simulink model "ModeAdjust"  (R2018b)
settings: Solver=FixedStepDiscrete  StartTime=0.0  StopTime=inf  FixedStep=0.01  RelTol=1e-3
undefined symbols (not defined in the file or in its folder): IfKeSMSbSeatMovBkRclnEnable_Val, IfKeSMSbSeatMovFrwdBkwdEnable_Val, IfKeSMSbSeatMovFtrstEnable_Val, IfKeSMSbSeatMovHdrstFrwdBkwdEnable_Val, IfKeSMSbSeatMovHdUpwdDnwdEnable_Val, IfKeSMSbSeatMovLgrstEnable_Val, IfKeSMSbSeatMovLtwdRtwdEnable_Val, IfVeSMSeStNumConfig, KeSMSbArmscreenMovEnable_Val, KeSMSbSeatMovLgrstExpdEnable_Val, KeSMSuFirstRwStBackPosDelta_Val, KeSMSuFirstRwStBackPosTolr_Val, KeSMSuFirstRwStCushFrntPosDelta_Val, KeSMSuFirstRwStCushFrntPosTolr_Val, KeSMSuFirstRwStCushRePosDelta_Val, KeSMSuFirstRwStCushRePosTolr_Val, KeSMSuFirstRwStFootrestPosDelta_Val, KeSMSuFirstRwStFootrestPosTolr_Val, KeSMSuFirstRwStFwdBkwdPosDelta_Val, KeSMSuFirstRwStFwdBkwdPosTolr_Val, KeSMSuMdMotFinshdTm_Val, KeSMSuMdRetryTm1_Val, KeSMSuModeReqDurgTm_Val, KeSMSuSecRwStArmTochPosDelta_Val, KeSMSuSecRwStArmTochPosTolr_Val, KeSMSuSecRwStBackPosDelta_Val, KeSMSuSecRwStBackPosTolr_Val, KeSMSuSecRwStFtrstUpwdDnwdPosDelta_Val, KeSMSuSecRwStFtrstUpwdDnwdPosTolr_Val, KeSMSuSecRwStFwdBkwdPosDelta_Val, KeSMSuSecRwStFwdBkwdPosTolr_Val, KeSMSuSecRwStHeadrestFwdBkwdPosDelta_Val, KeSMSuSecRwStHeadrestFwdBkwdPosTolr_Val, KeSMSuSecRwStHeadrestUpwdDwnwdPosDelta_Val, KeSMSuSecRwStHeadrestUpwdDwnwdPosTolr_Val, KeSMSuSecRwStLegrestInOutPosDelta_Val, KeSMSuSecRwStLegrestInOutPosTolr_Val, KeSMSuSecRwStLegrestUpwdDwnwdPosDelta_Val, KeSMSuSecRwStLegrestUpwdDwnwdPosTolr_Val, KeSMSuSecRwStLwdRwdPosDelta_Val, KeSMSuSecRwStLwdRwdPosTolr_Val, KeSMSuSecRwStVIPFtrstRefAngle_Val, KeSMSuThirdRwStFwdBkwdPosDelta_Val, KeSMSuThirdRwStFwdBkwdPosTolr_Val, KeSMSuThrdRwCushFoldPosDelta_Val, KeSMSuThrdRwCushFoldPosTolr_Val, KeSMSuThrdRwStBackPosDelta_Val, KeSMSuThrdRwStBackPosTolr_Val, KeSMSw4SLegrstCloseMdSecRwLtStFtrstUpwdDnwdPos_Val, KeSMSw4SLegrstCloseMdSecRwLtStFtrstUpwdDnwdPosMax_Val, KeSMSw4SLegrstCloseMdSecRwLtStFtrstUpwdDnwdPosMin_Val, KeSMSw4SLegrstCloseMdSecRwLtStLgrstOtwdInwdPos_Val, KeSMSw4SLegrstCloseMdSecRwLtStLgrstOtwdInwdPosMax_Val, KeSMSw4SLegrstCloseMdSecRwLtStLgrstOtwdInwdPosMin_Val, KeSMSw4SLegrstCloseMdSecRwLtStLgrstUpwdDnwdPos_Val, KeSMSw4SLegrstCloseMdSecRwLtStLgrstUpwdDnwdPosMax_Val, KeSMSw4SLegrstCloseMdSecRwLtStLgrstUpwdDnwdPosMin_Val, KeSMSw4SLegrstCloseMdSecRwRtStFtrstUpwdDnwdPos_Val, KeSMSw4SLegrstCloseMdSecRwRtStFtrstUpwdDnwdPosMax_Val, KeSMSw4SLegrstCloseMdSecRwRtStFtrstUpwdDnwdPosMin_Val ... (+1138)
libraries: Lib x401
(part 29 of 35)

== system ModeAdjust/ModeAdjustRunnable_sys/ModeAdjust/ArrivedAtTargetPosChk/Ly/R2Rt ==
  SecRwLtStsPoss : Inport
  ModeStCalib_2L : Inport  Port=2
  StConfig : Inport  Port=3
  SecRwLtStsPoss4s : Inport  Port=4
  StConfig4s : Inport  Port=5
  SecRwRtStPossV : Inport  Port=6
  PosV4s : Inport  Port=7
  Rt4sHightIndex : Inport  Port=8
  PosDeltaCalib : Inport  Port=9
  Bus Creator{,1..6} (7 alike) : BusCreator  Inputs=9
  Bus Selector : BusSelector  OutputSignals=IfVeSMSuSecRwRtStBkReclnUpwdDnwdPos_Val_read,IfVeSMSuSecRwRtStFrwdBkwdPos_Val_read,IfVeSMSuSecRwRtStHPassStUpwdDnwdPos_Val_read,IfVeSMSuSecRwRtStLgrstUpwdDnwdPos_Val_read,IfVeSMSuSecRwRtStLtwdRtwdPos_Val_read,SecRwRtStArmScrnPos_Val_read
  Bus Selector1 : BusSelector  OutputSignals=IfVeSMSuSecRwRtStLgrstOtwdInwdPos_Val_read,IfVeSMSuRrRtStFtUpwdDnwdPos_Val_read,IfVeSMSuSecRwRtStHdrstFrwdBkwdPos_Val_read
  Bus Selector2 : BusSelector  OutputSignals=BkReclnUpwdDnwdPosMax,BkReclnUpwdDnwdPosMin,LgrstUpwdPosMax,LgrstUpwdPosMin,FtrstUpwdDnwdPosMax,FtrstUpwdDnwdPosMin
  Bus Selector3 : BusSelector  OutputSignals=LyRSecRwRtSt
  Bus Selector4 : BusSelector  OutputSignals=BkReclnUpwdDnwdMovConfig,ArmTouchMovConfig,FrwdBkwdMovConfig,LgrstUpwdMovConfig,LtwdRtwdMovConfig
  Bus Selector5 : BusSelector  OutputSignals=LgrstExpdMovConfig,FtrstMovConfig,HdrstUpwdDnwdMovConfig,HdrstFrwdBkwdMovConfig
  Bus Selector6 : BusSelector  OutputSignals=IfVeSMSuSecRwRtStBkReclnUpwdDnwdPosV_Val_read,IfVeSMSuSecRwRtStFrwdBkwdPosV_Val_read,IfVeSMSuSecRwRtStHPassStUpwdDnwdPosV_Val_read,IfVeSMSuSecRwRtStLgrstUpwdDnwdPosV_Val_read,IfVeSMSuSecRwRtStLtwdRtwdPosV_Val_read,SecRwRtStArmScrnPosV_Val_read
  Bus Selector7 : BusSelector  OutputSignals=IfVeSMSuSecRwRtStLgrstOtwdInwdPosV_Val_read,IfVeSMSuRrRtStFtUpwdDnwdPosV_Val_read,IfVeSMSuSecRwRtStHdrstFrwdBkwdPosV_Val_read
  Bus Selector8 : BusSelector  OutputSignals=HdrstUpwdDnwdPosMax,HdrstUpwdDnwdPosMin,HdrstFrwdBkwdnwdPosMax,HdrstFrwdBkwdnwdPosMin,LgrstOtwdInwdPosMax,LgrstOtwdInwdPosMin
  Bus Selector9 : BusSelector  OutputSignals=KeSMSuSecRwStHeadrestFwdBkwdPosDelta_Val,KeSMSuSecRwStHeadrestUpwdDwnwdPosDelta_Val,KeSMSuSecRwStLegrestInOutPosDelta_Val,KeSMSuSecRwStFtrstUpwdDnwdPosDelta_Val,KeSMSuSecRwStBackPosDelta_Val,KeSMSuSecRwStLegrestUpwdDwnwdPosDelta_Val
  CheckAtPos{,1..5} (6 alike) : Lib/CheckAtPos  SystemSampleTime=-1
  Constant{1..12} (12 alike) : Constant  Value=0  OutDataTypeStr=boolean
  IsArrivedTarZone{,1..5} (6 alike) : Lib/CommonUsed/IniPosjudg/Subsystem2  SystemSampleTime=-1
  Logical Operator9 : Logic  Inputs=6  AllPortsSameDT=off  OutDataTypeStr=boolean
  Multiport Switch : MultiPortSwitch  DataPortOrder=Zero-based contiguous  Inputs=7  DiagnosticForDefault=None  zeroidx=on
  PA_KeSMSw4sLyingMDSecRwRtStHdrstFrwdBkwdnwdPosMax_160_Val : Constant  Value=KeSMSw4sLyingMDSecRwRtStHdrstFrwdBkwdnwdPosMax_160_Val
  PA_KeSMSw4sLyingMDSecRwRtStHdrstFrwdBkwdnwdPosMax_165_Val : Constant  Value=KeSMSw4sLyingMDSecRwRtStHdrstFrwdBkwdnwdPosMax_165_Val
  PA_KeSMSw4sLyingMDSecRwRtStHdrstFrwdBkwdnwdPosMax_170_Val : Constant  Value=KeSMSw4sLyingMDSecRwRtStHdrstFrwdBkwdnwdPosMax_170_Val
  PA_KeSMSw4sLyingMDSecRwRtStHdrstFrwdBkwdnwdPosMax_175_Val : Constant  Value=KeSMSw4sLyingMDSecRwRtStHdrstFrwdBkwdnwdPosMax_175_Val
  PA_KeSMSw4sLyingMDSecRwRtStHdrstFrwdBkwdnwdPosMax_180_Val : Constant  Value=KeSMSw4sLyingMDSecRwRtStHdrstFrwdBkwdnwdPosMax_180_Val
  PA_KeSMSw4sLyingMDSecRwRtStHdrstFrwdBkwdnwdPosMax_Below160_Val : Constant  Value=KeSMSw4sLyingMDSecRwRtStHdrstFrwdBkwdnwdPosMax_Below160_Val
  PA_KeSMSw4sLyingMDSecRwRtStHdrstFrwdBkwdnwdPosMax_Over180_Val : Constant  Value=KeSMSw4sLyingMDSecRwRtStHdrstFrwdBkwdnwdPosMax_Over180_Val
  PA_KeSMSw4sLyingMDSecRwRtStHdrstFrwdBkwdnwdPosMin_160_Val : Constant  Value=KeSMSw4sLyingMDSecRwRtStHdrstFrwdBkwdnwdPosMin_160_Val
  PA_KeSMSw4sLyingMDSecRwRtStHdrstFrwdBkwdnwdPosMin_165_Val : Constant  Value=KeSMSw4sLyingMDSecRwRtStHdrstFrwdBkwdnwdPosMin_165_Val
  PA_KeSMSw4sLyingMDSecRwRtStHdrstFrwdBkwdnwdPosMin_170_Val : Constant  Value=KeSMSw4sLyingMDSecRwRtStHdrstFrwdBkwdnwdPosMin_170_Val
  PA_KeSMSw4sLyingMDSecRwRtStHdrstFrwdBkwdnwdPosMin_175_Val : Constant  Value=KeSMSw4sLyingMDSecRwRtStHdrstFrwdBkwdnwdPosMin_175_Val
  PA_KeSMSw4sLyingMDSecRwRtStHdrstFrwdBkwdnwdPosMin_180_Val : Constant  Value=KeSMSw4sLyingMDSecRwRtStHdrstFrwdBkwdnwdPosMin_180_Val
  PA_KeSMSw4sLyingMDSecRwRtStHdrstFrwdBkwdnwdPosMin_Below160_Val : Constant  Value=KeSMSw4sLyingMDSecRwRtStHdrstFrwdBkwdnwdPosMin_Below160_Val
  PA_KeSMSw4sLyingMDSecRwRtStHdrstFrwdBkwdnwdPosMin_Over180_Val : Constant  Value=KeSMSw4sLyingMDSecRwRtStHdrstFrwdBkwdnwdPosMin_Over180_Val
  PA_KeSMSw4sLyingMDSecRwRtStHdrstFrwdBkwdnwdPos_160_Val : Constant  Value=KeSMSw4sLyingMDSecRwRtStHdrstFrwdBkwdnwdPos_160_Val
  PA_KeSMSw4sLyingMDSecRwRtStHdrstFrwdBkwdnwdPos_165_Val : Constant  Value=KeSMSw4sLyingMDSecRwRtStHdrstFrwdBkwdnwdPos_165_Val
  PA_KeSMSw4sLyingMDSecRwRtStHdrstFrwdBkwdnwdPos_170_Val : Constant  Value=KeSMSw4sLyingMDSecRwRtStHdrstFrwdBkwdnwdPos_170_Val
  PA_KeSMSw4sLyingMDSecRwRtStHdrstFrwdBkwdnwdPos_175_Val : Constant  Value=KeSMSw4sLyingMDSecRwRtStHdrstFrwdBkwdnwdPos_175_Val
  PA_KeSMSw4sLyingMDSecRwRtStHdrstFrwdBkwdnwdPos_180_Val : Constant  Value=KeSMSw4sLyingMDSecRwRtStHdrstFrwdBkwdnwdPos_180_Val
  PA_KeSMSw4sLyingMDSecRwRtStHdrstFrwdBkwdnwdPos_Below160_Val : Constant  Value=KeSMSw4sLyingMDSecRwRtStHdrstFrwdBkwdnwdPos_Below160_Val
  PA_KeSMSw4sLyingMDSecRwRtStHdrstFrwdBkwdnwdPos_Over180_Val : Constant  Value=KeSMSw4sLyingMDSecRwRtStHdrstFrwdBkwdnwdPos_Over180_Val
  PA_KeSMSw4sLyingMDSecRwRtStHdrstUpwdPosMax_160_Val : Constant  Value=KeSMSw4sLyingMDSecRwRtStHdrstUpwdPosMax_160_Val
  PA_KeSMSw4sLyingMDSecRwRtStHdrstUpwdPosMax_165_Val : Constant  Value=KeSMSw4sLyingMDSecRwRtStHdrstUpwdPosMax_165_Val
  PA_KeSMSw4sLyingMDSecRwRtStHdrstUpwdPosMax_170_Val : Constant  Value=KeSMSw4sLyingMDSecRwRtStHdrstUpwdPosMax_170_Val
  PA_KeSMSw4sLyingMDSecRwRtStHdrstUpwdPosMax_175_Val : Constant  Value=KeSMSw4sLyingMDSecRwRtStHdrstUpwdPosMax_175_Val
  PA_KeSMSw4sLyingMDSecRwRtStHdrstUpwdPosMax_180_Val : Constant  Value=KeSMSw4sLyingMDSecRwRtStHdrstUpwdPosMax_180_Val
  PA_KeSMSw4sLyingMDSecRwRtStHdrstUpwdPosMax_Below160_Val : Constant  Value=KeSMSw4sLyingMDSecRwRtStHdrstUpwdPosMax_Below160_Val
  PA_KeSMSw4sLyingMDSecRwRtStHdrstUpwdPosMax_Over180_Val : Constant  Value=KeSMSw4sLyingMDSecRwRtStHdrstUpwdPosMax_Over180_Val
  PA_KeSMSw4sLyingMDSecRwRtStHdrstUpwdPosMin_160_Val : Constant  Value=KeSMSw4sLyingMDSecRwRtStHdrstUpwdPosMin_160_Val
  PA_KeSMSw4sLyingMDSecRwRtStHdrstUpwdPosMin_165_Val : Constant  Value=KeSMSw4sLyingMDSecRwRtStHdrstUpwdPosMin_165_Val
  PA_KeSMSw4sLyingMDSecRwRtStHdrstUpwdPosMin_170_Val : Constant  Value=KeSMSw4sLyingMDSecRwRtStHdrstUpwdPosMin_170_Val
  PA_KeSMSw4sLyingMDSecRwRtStHdrstUpwdPosMin_175_Val : Constant  Value=KeSMSw4sLyingMDSecRwRtStHdrstUpwdPosMin_175_Val
  PA_KeSMSw4sLyingMDSecRwRtStHdrstUpwdPosMin_180_Val : Constant  Value=KeSMSw4sLyingMDSecRwRtStHdrstUpwdPosMin_180_Val
  PA_KeSMSw4sLyingMDSecRwRtStHdrstUpwdPosMin_Below160_Val : Constant  Value=KeSMSw4sLyingMDSecRwRtStHdrstUpwdPosMin_Below160_Val
  PA_KeSMSw4sLyingMDSecRwRtStHdrstUpwdPosMin_Over180_Val : Constant  Value=KeSMSw4sLyingMDSecRwRtStHdrstUpwdPosMin_Over180_Val
  PA_KeSMSw4sLyingMDSecRwRtStHdrstUpwdPos_160_Val : Constant  Value=KeSMSw4sLyingMDSecRwRtStHdrstUpwdPos_160_Val
  PA_KeSMSw4sLyingMDSecRwRtStHdrstUpwdPos_165_Val : Constant  Value=KeSMSw4sLyingMDSecRwRtStHdrstUpwdPos_165_Val
  PA_KeSMSw4sLyingMDSecRwRtStHdrstUpwdPos_170_Val : Constant  Value=KeSMSw4sLyingMDSecRwRtStHdrstUpwdPos_170_Val
  PA_KeSMSw4sLyingMDSecRwRtStHdrstUpwdPos_175_Val : Constant  Value=KeSMSw4sLyingMDSecRwRtStHdrstUpwdPos_175_Val
  PA_KeSMSw4sLyingMDSecRwRtStHdrstUpwdPos_180_Val : Constant  Value=KeSMSw4sLyingMDSecRwRtStHdrstUpwdPos_180_Val
  PA_KeSMSw4sLyingMDSecRwRtStHdrstUpwdPos_Below160_Val : Constant  Value=KeSMSw4sLyingMDSecRwRtStHdrstUpwdPos_Below160_Val
  PA_KeSMSw4sLyingMDSecRwRtStHdrstUpwdPos_Over180_Val : Constant  Value=KeSMSw4sLyingMDSecRwRtStHdrstUpwdPos_Over180_Val
  PA_KeSMSw4sLyingMDSecRwRtStLgrstOtwdInwdPosMax_160_Val : Constant  Value=KeSMSw4sLyingMDSecRwRtStLgrstOtwdInwdPosMax_160_Val
  PA_KeSMSw4sLyingMDSecRwRtStLgrstOtwdInwdPosMax_165_Val : Constant  Value=KeSMSw4sLyingMDSecRwRtStLgrstOtwdInwdPosMax_165_Val
  PA_KeSMSw4sLyingMDSecRwRtStLgrstOtwdInwdPosMax_170_Val : Constant  Value=KeSMSw4sLyingMDSecRwRtStLgrstOtwdInwdPosMax_170_Val
  PA_KeSMSw4sLyingMDSecRwRtStLgrstOtwdInwdPosMax_175_Val : Constant  Value=KeSMSw4sLyingMDSecRwRtStLgrstOtwdInwdPosMax_175_Val
  PA_KeSMSw4sLyingMDSecRwRtStLgrstOtwdInwdPosMax_180_Val : Constant  Value=KeSMSw4sLyingMDSecRwRtStLgrstOtwdInwdPosMax_180_Val
  PA_KeSMSw4sLyingMDSecRwRtStLgrstOtwdInwdPosMax_Below160_Val : Constant  Value=KeSMSw4sLyingMDSecRwRtStLgrstOtwdInwdPosMax_Below160_Val
  PA_KeSMSw4sLyingMDSecRwRtStLgrstOtwdInwdPosMax_Over180_Val : Constant  Value=KeSMSw4sLyingMDSecRwRtStLgrstOtwdInwdPosMax_Over180_Val
  PA_KeSMSw4sLyingMDSecRwRtStLgrstOtwdInwdPosMin_160_Val : Constant  Value=KeSMSw4sLyingMDSecRwRtStLgrstOtwdInwdPosMin_160_Val
  PA_KeSMSw4sLyingMDSecRwRtStLgrstOtwdInwdPosMin_165_Val : Constant  Value=KeSMSw4sLyingMDSecRwRtStLgrstOtwdInwdPosMin_165_Val
  PA_KeSMSw4sLyingMDSecRwRtStLgrstOtwdInwdPosMin_170_Val : Constant  Value=KeSMSw4sLyingMDSecRwRtStLgrstOtwdInwdPosMin_170_Val
  PA_KeSMSw4sLyingMDSecRwRtStLgrstOtwdInwdPosMin_175_Val : Constant  Value=KeSMSw4sLyingMDSecRwRtStLgrstOtwdInwdPosMin_175_Val
  PA_KeSMSw4sLyingMDSecRwRtStLgrstOtwdInwdPosMin_180_Val : Constant  Value=KeSMSw4sLyingMDSecRwRtStLgrstOtwdInwdPosMin_180_Val
  PA_KeSMSw4sLyingMDSecRwRtStLgrstOtwdInwdPosMin_Below160_Val : Constant  Value=KeSMSw4sLyingMDSecRwRtStLgrstOtwdInwdPosMin_Below160_Val
  PA_KeSMSw4sLyingMDSecRwRtStLgrstOtwdInwdPosMin_Over180_Val : Constant  Value=KeSMSw4sLyingMDSecRwRtStLgrstOtwdInwdPosMin_Over180_Val
  PA_KeSMSw4sLyingMDSecRwRtStLgrstOtwdInwdPos_160_Val : Constant  Value=KeSMSw4sLyingMDSecRwRtStLgrstOtwdInwdPos_160_Val
  PA_KeSMSw4sLyingMDSecRwRtStLgrstOtwdInwdPos_165_Val : Constant  Value=KeSMSw4sLyingMDSecRwRtStLgrstOtwdInwdPos_165_Val
  PA_KeSMSw4sLyingMDSecRwRtStLgrstOtwdInwdPos_170_Val : Constant  Value=KeSMSw4sLyingMDSecRwRtStLgrstOtwdInwdPos_170_Val
  PA_KeSMSw4sLyingMDSecRwRtStLgrstOtwdInwdPos_175_Val : Constant  Value=KeSMSw4sLyingMDSecRwRtStLgrstOtwdInwdPos_175_Val
  PA_KeSMSw4sLyingMDSecRwRtStLgrstOtwdInwdPos_180_Val : Constant  Value=KeSMSw4sLyingMDSecRwRtStLgrstOtwdInwdPos_180_Val
  PA_KeSMSw4sLyingMDSecRwRtStLgrstOtwdInwdPos_Below160_Val : Constant  Value=KeSMSw4sLyingMDSecRwRtStLgrstOtwdInwdPos_Below160_Val
  PA_KeSMSw4sLyingMDSecRwRtStLgrstOtwdInwdPos_Over180_Val : Constant  Value=KeSMSw4sLyingMDSecRwRtStLgrstOtwdInwdPos_Over180_Val
  R2Lt_ArrivedTarPos : Outport
  Calib_Ly4sRAdpt : Outport  Port=2
  wires:
  Bus Selector5/2 -> [FtrstMovConfig]  "<FtrstMovConfig>"
  Bus Selector5/1 -> [LgrstExpdMovConfig]  "<LgrstExpdMovConfig>"
  Bus Selector5/3 -> [HdrstMovConfig]  "<HdrstUpwdDnwdMovConfig>"
  StConfig4s/1 -> Bus Selector5/1
  IsArrivedTarZone4/1 -> [Step1_5_ArrivedTarPos]
  [KeSMSuSecRwStLegrestInOutPosDelta_Val] -> IsArrivedTarZone4/3
  [SecRwLtStLgrstOtwdInwdPos] -> IsArrivedTarZone4/1
  [K_LgrstOtwdInwdPos_Max] -> IsArrivedTarZone4/4
  [K_LgrstOtwdInwdPos_Min] -> IsArrivedTarZone4/2
  IsArrivedTarZone3/1 -> [Step1_4_ArrivedTarPos]
  [K_FtrstUpwdDnwdPos_Max] -> IsArrivedTarZone3/4
  [K_FtrstUpwdDnwdPos_Min] -> IsArrivedTarZone3/2
  Bus Selector2/6 -> [K_FtrstUpwdDnwdPos_Min]  "<FtrstUpwdDnwdPosMin>"
  Bus Selector2/5 -> [K_FtrstUpwdDnwdPos_Max]  "<FtrstUpwdDnwdPosMax>"
  [IfVeSMSuRrLtStFtUpwdDnwdPos] -> IsArrivedTarZone3/1
  Bus Selector1/2 -> [IfVeSMSuRrLtStFtUpwdDnwdPos]  "<IfVeSMSuRrRtStFtUpwdDnwdPos_Val_read>"
  Bus Selector1/1 -> [SecRwLtStLgrstOtwdInwdPos]  "<IfVeSMSuSecRwRtStLgrstOtwdInwdPos_Val_read>"
  SecRwLtStsPoss4s/1 -> Bus Selector1/1
  [KeSMSuSecRwStFtrstUpwdDnwdPosDelta_Val] -> IsArrivedTarZone3/3
  [KeSMSuSecRwStHeadrestUpwdDwnwdPosDelta_Val] -> IsArrivedTarZone2/3
  [SecRwLtStHPassStUpwdDnwdPos] -> IsArrivedTarZone2/1
  [K_HdrstUpwdPosMin] -> IsArrivedTarZone2/2
  [K_HdrstUpwdPosMax] -> IsArrivedTarZone2/4
  Bus Selector4/1 -> [BkReclnUpwdDnwdMovConfig]  "<BkReclnUpwdDnwdMovConfig>"
  Bus Selector4/2 -> [ArmTouchMovConfig]  "<ArmTouchMovConfig>"
  Bus Selector4/4 -> [LgrstUpwdMovConfig]  "<LgrstUpwdMovConfig>"
  Bus Selector4/5 -> [LtwdRtwdMovConfig]  "<LtwdRtwdMovConfig>"
  Bus Selector4/3 -> [FrwdBkwdMovConfig]  "<FrwdBkwdMovConfig>"
  StConfig/1 -> Bus Selector4/1
  ModeStCalib_2L/1 -> Bus Selector3/1
  Bus Selector2/2 -> [K_BkReclnUpwdDnwdPosMin]  "<BkReclnUpwdDnwdPosMin>"
  Bus Selector3/1 -> Bus Selector2/1  "<LyRSecRwRtSt>"
  Bus Selector2/1 -> [K_BkReclnUpwdDnwdPosMax]  "<BkReclnUpwdDnwdPosMax>"
  Bus Selector2/3 -> [K_LgrstUpwdPosMax]  "<LgrstUpwdPosMax>"
  Bus Selector2/4 -> [K_LgrstUpwdPosMin]  "<LgrstUpwdPosMin>"
  [KeSMSuSecRwStLegrestUpwdDwnwdPosDelta_Val] -> IsArrivedTarZone1/3
  [K_LgrstUpwdPosMax] -> IsArrivedTarZone1/4
  [K_BkReclnUpwdDnwdPosMax] -> IsArrivedTarZone/4
  [KeSMSuSecRwStBackPosDelta_Val] -> IsArrivedTarZone/3
  Bus Selector/6 -> [SecRwLtStArmScrnPos]  "<SecRwRtStArmScrnPos_Val_read>"
  IsArrivedTarZone2/1 -> [Step1_3_ArrivedTarPos]
  Logical Operator9/1 -> R2Lt_ArrivedTarPos/1
  IsArrivedTarZone1/1 -> [Step1_2_ArrivedTarPos]
  [SecRwLtStLgrstUpwdDnwdPos] -> IsArrivedTarZone1/1
  [K_LgrstUpwdPosMin] -> IsArrivedTarZone1/2
  Bus Selector/1 -> [SecRwLtStBkReclnUpwdDnwdPos]  "<IfVeSMSuSecRwRtStBkReclnUpwdDnwdPos_Val_read>"
  Bus Selector/2 -> [SecRwLtStFrwdBkwdPos]  "<IfVeSMSuSecRwRtStFrwdBkwdPos_Val_read>"
  Bus Selector/4 -> [SecRwLtStLgrstUpwdDnwdPos]  "<IfVeSMSuSecRwRtStLgrstUpwdDnwdPos_Val_read>"
  Bus Selector/3 -> [SecRwLtStHPassStUpwdDnwdPos]  "<IfVeSMSuSecRwRtStHPassStUpwdDnwdPos_Val_read>"
  SecRwLtStsPoss/1 -> Bus Selector/1
  Bus Selector/5 -> [SecRwLtStLtwdRtwdPos]  "<IfVeSMSuSecRwRtStLtwdRtwdPos_Val_read>"
  [K_BkReclnUpwdDnwdPosMin] -> IsArrivedTarZone/2
  [SecRwLtStBkReclnUpwdDnwdPos] -> IsArrivedTarZone/1
  IsArrivedTarZone/1 -> [Step1_1_ArrivedTarPos]
  Bus Selector6/1 -> [SecRwRtStBkReclnUpwdDnwdPosV]  "<IfVeSMSuSecRwRtStBkReclnUpwdDnwdPosV_Val_read>"
  Bus Selector6/3 -> [SecRwRtStHPassStUpwdDnwdPosV]  "<IfVeSMSuSecRwRtStHPassStUpwdDnwdPosV_Val_read>"
  Bus Selector6/2 -> [SecRwRtStFrwdBkwdPosV]  "<IfVeSMSuSecRwRtStFrwdBkwdPosV_Val_read>"
  Bus Selector6/5 -> [SecRwRtStLtwdRtwdPosV]  "<IfVeSMSuSecRwRtStLtwdRtwdPosV_Val_read>"
  SecRwRtStPossV/1 -> Bus Selector6/1
  Bus Selector6/4 -> [SecRwRtStLgrstUpwdDnwdPosV]  "<IfVeSMSuSecRwRtStLgrstUpwdDnwdPosV_Val_read>"
  Bus Selector6/6 -> [SecRwRtStArmScrnPosV]  "<SecRwRtStArmScrnPosV_Val_read>"
  Bus Selector7/1 -> [SecRwLtStLgrstOtwdInwdPosV]  "<IfVeSMSuSecRwRtStLgrstOtwdInwdPosV_Val_read>"
  Bus Selector7/2 -> [RrLtStFtUpwdDnwdPosV]  "<IfVeSMSuRrRtStFtUpwdDnwdPosV_Val_read>"
  PosV4s/1 -> Bus Selector7/1
  [BkReclnUpwdDnwdMovConfig] -> CheckAtPos/1
  [Step1_1_ArrivedTarPos] -> CheckAtPos/3
  [LgrstUpwdMovConfig] -> CheckAtPos1/1
  [Step1_2_ArrivedTarPos] -> CheckAtPos1/3
  [HdrstMovConfig] -> CheckAtPos2/1
  [Step1_3_ArrivedTarPos] -> CheckAtPos2/3
  [FtrstMovConfig] -> CheckAtPos3/1
  [Step1_4_ArrivedTarPos] -> CheckAtPos3/3
  [LgrstExpdMovConfig] -> CheckAtPos4/1
  [Step1_5_ArrivedTarPos] -> CheckAtPos4/3
  [SecRwRtStBkReclnUpwdDnwdPosV] -> CheckAtPos/2
  [SecRwRtStHPassStUpwdDnwdPosV] -> CheckAtPos2/2
  [RrLtStFtUpwdDnwdPosV] -> CheckAtPos3/2
  [SecRwLtStLgrstOtwdInwdPosV] -> CheckAtPos4/2
  [SecRwRtStLgrstUpwdDnwdPosV] -> CheckAtPos1/2
  CheckAtPos2/1 -> Logical Operator9/3  "LyR_Step1_3_ArrivedTarPos"
  CheckAtPos1/1 -> Logical Operator9/2  "LyR_Step1_2_ArrivedTarPos"
  CheckAtPos3/1 -> Logical Operator9/4  "LyR_Step1_4_ArrivedTarPos"
  CheckAtPos/1 -> Logical Operator9/1  "LyR_Step1_1_ArrivedTarPos"
  CheckAtPos4/1 -> Logical Operator9/5  "LyR_Step1_5_ArrivedTarPos"
  Constant9/1 -> CheckAtPos/4
  Constant10/1 -> CheckAtPos/5
  Constant2/1 -> CheckAtPos1/4
  Constant1/1 -> CheckAtPos1/5
  Constant4/1 -> CheckAtPos2/4
  Constant3/1 -> CheckAtPos2/5
  Constant6/1 -> CheckAtPos3/4
  Constant5/1 -> CheckAtPos3/5
  Constant8/1 -> CheckAtPos4/4
  Constant7/1 -> CheckAtPos4/5
  [SecRwRtStHdrstFrwdBkwdPos] -> IsArrivedTarZone5/1
  [K_HdrstFrwdBkwdnwdPosMax] -> IsArrivedTarZone5/4
  [K_HdrstFrwdBkwdnwdPosMin] -> IsArrivedTarZone5/2
  [KeSMSuSecRwStHeadrestFwdBkwdPosDelta_Val] -> IsArrivedTarZone5/3
  IsArrivedTarZone5/1 -> [Step1_6_ArrivedTarPos]
  [Step1_6_ArrivedTarPos] -> CheckAtPos5/3
  [SecRwRtStHdrstFrwdBkwdPosV] -> CheckAtPos5/2
  Constant12/1 -> CheckAtPos5/4
  Constant11/1 -> CheckAtPos5/5
  CheckAtPos5/1 -> Logical Operator9/6  "LyR_Step1_6_ArrivedTarPos"
  [HdrstFrwdBkwdMovConfig] -> CheckAtPos5/1
  Bus Selector5/4 -> [HdrstFrwdBkwdMovConfig]  "<HdrstFrwdBkwdMovConfig>"
  Bus Selector7/3 -> [SecRwRtStHdrstFrwdBkwdPosV]  "<IfVeSMSuSecRwRtStHdrstFrwdBkwdPosV_Val_read>"
  Bus Selector1/3 -> [SecRwRtStHdrstFrwdBkwdPos]  "<IfVeSMSuSecRwRtStHdrstFrwdBkwdPos_Val_read>"
  PA_KeSMSw4sLyingMDSecRwRtStLgrstOtwdInwdPos_Over180_Val/1 -> Bus Creator6/4  "LgrstOtwdInwdPos"
  PA_KeSMSw4sLyingMDSecRwRtStHdrstFrwdBkwdnwdPosMin_180_Val/1 -> Bus Creator5/9  "HdrstFrwdBkwdnwdPosMin"
  PA_KeSMSw4sLyingMDSecRwRtStHdrstFrwdBkwdnwdPosMax_180_Val/1 -> Bus Creator5/8  "HdrstFrwdBkwdnwdPosMax"
  PA_KeSMSw4sLyingMDSecRwRtStLgrstOtwdInwdPos_Below160_Val/1 -> Bus Creator/4  "LgrstOtwdInwdPos"
  PA_KeSMSw4sLyingMDSecRwRtStLgrstOtwdInwdPosMax_Below160_Val/1 -> Bus Creator/5  "LgrstOtwdInwdPosMax"
  PA_KeSMSw4sLyingMDSecRwRtStLgrstOtwdInwdPos_170_Val/1 -> Bus Creator3/4  "LgrstOtwdInwdPos"
  PA_KeSMSw4sLyingMDSecRwRtStLgrstOtwdInwdPosMax_170_Val/1 -> Bus Creator3/5  "LgrstOtwdInwdPosMax"
  PA_KeSMSw4sLyingMDSecRwRtStHdrstUpwdPosMin_170_Val/1 -> Bus Creator3/3  "HdrstUpwdDnwdPosMin"
  PA_KeSMSw4sLyingMDSecRwRtStLgrstOtwdInwdPosMin_175_Val/1 -> Bus Creator4/6  "LgrstOtwdInwdPosMin"
  PA_KeSMSw4sLyingMDSecRwRtStHdrstFrwdBkwdnwdPosMin_175_Val/1 -> Bus Creator4/9  "HdrstFrwdBkwdnwdPosMin"
  PA_KeSMSw4sLyingMDSecRwRtStLgrstOtwdInwdPosMin_Below160_Val/1 -> Bus Creator/6  "LgrstOtwdInwdPosMin"
  PA_KeSMSw4sLyingMDSecRwRtStHdrstFrwdBkwdnwdPos_160_Val/1 -> Bus Creator1/7  "HdrstFrwdBkwdnwdPos"
  PA_KeSMSw4sLyingMDSecRwRtStHdrstUpwdPosMin_165_Val/1 -> Bus Creator2/3  "HdrstUpwdDnwdPosMin"
  PA_KeSMSw4sLyingMDSecRwRtStHdrstFrwdBkwdnwdPosMax_160_Val/1 -> Bus Creator1/8  "HdrstFrwdBkwdnwdPosMax"
  PA_KeSMSw4sLyingMDSecRwRtStLgrstOtwdInwdPos_165_Val/1 -> Bus Creator2/4  "LgrstOtwdInwdPos"
  PA_KeSMSw4sLyingMDSecRwRtStHdrstUpwdPos_Below160_Val/1 -> Bus Creator/1  "HdrstUpwdDnwdPos"
  PA_KeSMSw4sLyingMDSecRwRtStLgrstOtwdInwdPosMax_165_Val/1 -> Bus Creator2/5  "LgrstOtwdInwdPosMax"
  PA_KeSMSw4sLyingMDSecRwRtStLgrstOtwdInwdPosMin_180_Val/1 -> Bus Creator5/6  "LgrstOtwdInwdPosMin"
  PA_KeSMSw4sLyingMDSecRwRtStLgrstOtwdInwdPosMax_180_Val/1 -> Bus Creator5/5  "LgrstOtwdInwdPosMax"
  PA_KeSMSw4sLyingMDSecRwRtStHdrstUpwdPosMin_Below160_Val/1 -> Bus Creator/3  "HdrstUpwdDnwdPosMin"
  PA_KeSMSw4sLyingMDSecRwRtStHdrstUpwdPosMin_175_Val/1 -> Bus Creator4/3  "HdrstUpwdDnwdPosMin"
  PA_KeSMSw4sLyingMDSecRwRtStHdrstFrwdBkwdnwdPos_180_Val/1 -> Bus Creator5/7  "HdrstFrwdBkwdnwdPos"
  PA_KeSMSw4sLyingMDSecRwRtStHdrstFrwdBkwdnwdPos_Over180_Val/1 -> Bus Creator6/7  "HdrstFrwdBkwdnwdPos"
  PA_KeSMSw4sLyingMDSecRwRtStHdrstUpwdPosMax_180_Val/1 -> Bus Creator5/2  "HdrstUpwdDnwdPosMax"
  PA_KeSMSw4sLyingMDSecRwRtStHdrstFrwdBkwdnwdPosMax_Over180_Val/1 -> Bus Creator6/8  "HdrstFrwdBkwdnwdPosMax"
  PA_KeSMSw4sLyingMDSecRwRtStHdrstFrwdBkwdnwdPosMax_175_Val/1 -> Bus Creator4/8  "HdrstFrwdBkwdnwdPosMax"
  PA_KeSMSw4sLyingMDSecRwRtStHdrstFrwdBkwdnwdPosMax_165_Val/1 -> Bus Creator2/8  "HdrstFrwdBkwdnwdPosMax"
  PA_KeSMSw4sLyingMDSecRwRtStHdrstUpwdPosMax_165_Val/1 -> Bus Creator2/2  "HdrstUpwdDnwdPosMax"
  PA_KeSMSw4sLyingMDSecRwRtStHdrstFrwdBkwdnwdPos_175_Val/1 -> Bus Creator4/7  "HdrstFrwdBkwdnwdPos"
  PA_KeSMSw4sLyingMDSecRwRtStHdrstUpwdPos_160_Val/1 -> Bus Creator1/1  "HdrstUpwdDnwdPos"
  PA_KeSMSw4sLyingMDSecRwRtStLgrstOtwdInwdPosMin_Over180_Val/1 -> Bus Creator6/6  "LgrstOtwdInwdPosMin"
  PA_KeSMSw4sLyingMDSecRwRtStLgrstOtwdInwdPos_160_Val/1 -> Bus Creator1/4  "LgrstOtwdInwdPos"
  PA_KeSMSw4sLyingMDSecRwRtStHdrstUpwdPos_170_Val/1 -> Bus Creator3/1  "HdrstUpwdDnwdPos"
  PA_KeSMSw4sLyingMDSecRwRtStLgrstOtwdInwdPosMax_Over180_Val/1 -> Bus Creator6/5  "LgrstOtwdInwdPosMax"
  PA_KeSMSw4sLyingMDSecRwRtStHdrstFrwdBkwdnwdPos_Below160_Val/1 -> Bus Creator/7  "HdrstFrwdBkwdnwdPos"
  PA_KeSMSw4sLyingMDSecRwRtStLgrstOtwdInwdPosMax_175_Val/1 -> Bus Creator4/5  "LgrstOtwdInwdPosMax"
  PA_KeSMSw4sLyingMDSecRwRtStLgrstOtwdInwdPosMin_160_Val/1 -> Bus Creator1/6  "LgrstOtwdInwdPosMin"
  PA_KeSMSw4sLyingMDSecRwRtStHdrstUpwdPos_165_Val/1 -> Bus Creator2/1  "HdrstUpwdDnwdPos"
  Bus Creator3/1 -> Multiport Switch/5  "Ly4sRAdpt"
  Bus Creator6/1 -> Multiport Switch/8  "Ly4sRAdpt"
  Bus Creator2/1 -> Multiport Switch/4  "Ly4sRAdpt"
  Bus Creator4/1 -> Multiport Switch/6  "Ly4sRAdpt"
  PA_KeSMSw4sLyingMDSecRwRtStHdrstUpwdPosMin_180_Val/1 -> Bus Creator5/3  "HdrstUpwdDnwdPosMin"
  Bus Creator1/1 -> Multiport Switch/3  "Ly4sRAdpt"
  PA_KeSMSw4sLyingMDSecRwRtStHdrstUpwdPos_Over180_Val/1 -> Bus Creator6/1  "HdrstUpwdDnwdPos"
  PA_KeSMSw4sLyingMDSecRwRtStHdrstUpwdPosMin_Over180_Val/1 -> Bus Creator6/3  "HdrstUpwdDnwdPosMin"
  PA_KeSMSw4sLyingMDSecRwRtStHdrstFrwdBkwdnwdPosMin_Below160_Val/1 -> Bus Creator/9  "HdrstFrwdBkwdnwdPosMin"
  PA_KeSMSw4sLyingMDSecRwRtStHdrstUpwdPosMin_160_Val/1 -> Bus Creator1/3  "HdrstUpwdDnwdPosMin"
  PA_KeSMSw4sLyingMDSecRwRtStHdrstUpwdPosMax_Over180_Val/1 -> Bus Creator6/2  "HdrstUpwdDnwdPosMax"
  PA_KeSMSw4sLyingMDSecRwRtStHdrstFrwdBkwdnwdPosMin_160_Val/1 -> Bus Creator1/9  "HdrstFrwdBkwdnwdPosMin"
  Bus Creator5/1 -> Multiport Switch/7  "Ly4sRAdpt"
  Rt4sHightIndex/1 -> Multiport Switch/1
  Bus Creator/1 -> Multiport Switch/2  "Ly4sRAdpt"
  PA_KeSMSw4sLyingMDSecRwRtStHdrstUpwdPosMax_160_Val/1 -> Bus Creator1/2  "HdrstUpwdDnwdPosMax"
  PA_KeSMSw4sLyingMDSecRwRtStHdrstUpwdPos_175_Val/1 -> Bus Creator4/1  "HdrstUpwdDnwdPos"
  PA_KeSMSw4sLyingMDSecRwRtStHdrstFrwdBkwdnwdPosMax_Below160_Val/1 -> Bus Creator/8  "HdrstFrwdBkwdnwdPosMax"
  PA_KeSMSw4sLyingMDSecRwRtStHdrstUpwdPosMax_Below160_Val/1 -> Bus Creator/2  "HdrstUpwdDnwdPosMax"
  PA_KeSMSw4sLyingMDSecRwRtStLgrstOtwdInwdPosMax_160_Val/1 -> Bus Creator1/5  "LgrstOtwdInwdPosMax"
  PA_KeSMSw4sLyingMDSecRwRtStHdrstUpwdPos_180_Val/1 -> Bus Creator5/1  "HdrstUpwdDnwdPos"
  PA_KeSMSw4sLyingMDSecRwRtStLgrstOtwdInwdPos_180_Val/1 -> Bus Creator5/4  "LgrstOtwdInwdPos"
  PA_KeSMSw4sLyingMDSecRwRtStHdrstFrwdBkwdnwdPos_170_Val/1 -> Bus Creator3/7  "HdrstFrwdBkwdnwdPos"
  PA_KeSMSw4sLyingMDSecRwRtStHdrstFrwdBkwdnwdPos_165_Val/1 -> Bus Creator2/7  "HdrstFrwdBkwdnwdPos"
  PA_KeSMSw4sLyingMDSecRwRtStLgrstOtwdInwdPosMin_165_Val/1 -> Bus Creator2/6  "LgrstOtwdInwdPosMin"
  PA_KeSMSw4sLyingMDSecRwRtStLgrstOtwdInwdPos_175_Val/1 -> Bus Creator4/4  "LgrstOtwdInwdPos"
  PA_KeSMSw4sLyingMDSecRwRtStLgrstOtwdInwdPosMin_170_Val/1 -> Bus Creator3/6  "LgrstOtwdInwdPosMin"
  PA_KeSMSw4sLyingMDSecRwRtStHdrstFrwdBkwdnwdPosMin_170_Val/1 -> Bus Creator3/9  "HdrstFrwdBkwdnwdPosMin"
  PA_KeSMSw4sLyingMDSecRwRtStHdrstFrwdBkwdnwdPosMin_Over180_Val/1 -> Bus Creator6/9  "HdrstFrwdBkwdnwdPosMin"
  PA_KeSMSw4sLyingMDSecRwRtStHdrstUpwdPosMax_175_Val/1 -> Bus Creator4/2  "HdrstUpwdDnwdPosMax"
  PA_KeSMSw4sLyingMDSecRwRtStHdrstFrwdBkwdnwdPosMax_170_Val/1 -> Bus Creator3/8  "HdrstFrwdBkwdnwdPosMax"
  PA_KeSMSw4sLyingMDSecRwRtStHdrstFrwdBkwdnwdPosMin_165_Val/1 -> Bus Creator2/9  "HdrstFrwdBkwdnwdPosMin"
  PA_KeSMSw4sLyingMDSecRwRtStHdrstUpwdPosMax_170_Val/1 -> Bus Creator3/2  "HdrstUpwdDnwdPosMax"
  Bus Selector8/5 -> [K_LgrstOtwdInwdPos_Max]  "<LgrstOtwdInwdPosMax>"
  Bus Selector8/6 -> [K_LgrstOtwdInwdPos_Min]  "<LgrstOtwdInwdPosMin>"
  Bus Selector8/1 -> [K_HdrstUpwdPosMax]  "<HdrstUpwdDnwdPosMax>"
  Bus Selector8/4 -> [K_HdrstFrwdBkwdnwdPosMin]  "<HdrstFrwdBkwdnwdPosMin>"
  Multiport Switch/1 -> Calib_Ly4sRAdpt/1, Bus Selector8/1
  Bus Selector8/2 -> [K_HdrstUpwdPosMin]  "<HdrstUpwdDnwdPosMin>"
  Bus Selector8/3 -> [K_HdrstFrwdBkwdnwdPosMax]  "<HdrstFrwdBkwdnwdPosMax>"
  Bus Selector9/5 -> [KeSMSuSecRwStBackPosDelta_Val]  "<KeSMSuSecRwStBackPosDelta_Val>"
  Bus Selector9/4 -> [KeSMSuSecRwStFtrstUpwdDnwdPosDelta_Val]  "<KeSMSuSecRwStFtrstUpwdDnwdPosDelta_Val>"
  Bus Selector9/6 -> [KeSMSuSecRwStLegrestUpwdDwnwdPosDelta_Val]  "<KeSMSuSecRwStLegrestUpwdDwnwdPosDelta_Val>"
  Bus Selector9/2 -> [KeSMSuSecRwStHeadrestUpwdDwnwdPosDelta_Val]  "<KeSMSuSecRwStHeadrestUpwdDwnwdPosDelta_Val>"
  Bus Selector9/3 -> [KeSMSuSecRwStLegrestInOutPosDelta_Val]  "<KeSMSuSecRwStLegrestInOutPosDelta_Val>"
  Bus Selector9/1 -> [KeSMSuSecRwStHeadrestFwdBkwdPosDelta_Val]  "<KeSMSuSecRwStHeadrestFwdBkwdPosDelta_Val>"
  PosDeltaCalib/1 -> Bus Selector9/1

== system ModeAdjust/ModeAdjustRunnable_sys/ModeAdjust/ArrivedAtTargetPosChk/Recovery/Drv ==
  DrvCurPos : Inport
  ModeStCalib_Drv : Inport  Port=2
  StConfig : Inport  Port=3
  DrvCurPosV : Inport  Port=4
  PosDeltaCalib : Inport  Port=5
  Bus Selector : BusSelector  OutputSignals=IfVeSMSuDrvStFtUpwdDnwdPos_Val_read,IfVeSMSuDrvStBkReclnUpwdDnwdPos_Val_read,IfVeSMSuDrvStCshnFrntUpwdDnwdPos_Val_read,IfVeSMSuDrvStCshnRrUpwdDnwdPos_Val_read,IfVeSMSuDrvStFrwdBkwdPos_Val_read
  Bus Selector1 : BusSelector  OutputSignals=IfVeSMSuDrvStFtUpwdDnwdPosV_Val_read,IfVeSMSuDrvStBkReclnUpwdDnwdPosV_Val_read,IfVeSMSuDrvStCshnFrntUpwdDnwdPosV_Val_read,IfVeSMSuDrvStCshnRrUpwdDnwdPosV_Val_read,IfVeSMSuDrvStFrwdBkwdPosV_Val_read
  Bus Selector2 : BusSelector  OutputSignals=BkReclnUpwdDnwdPos,BkReclnUpwdDnwdPosMax,BkReclnUpwdDnwdPosMin,FrwdBkwdPos,FrwdBkwdPosMax,FrwdBkwdPosMin,FtUpwdDnwdPos,FtUpwdDnwdPosMax,FtUpwdDnwdPosMin
  Bus Selector3 : BusSelector  OutputSignals=RecvDrvSt
  Bus Selector4 : BusSelector  OutputSignals=BkReclnUpwdDnwdMovConfig,FrwdBkwdMovConfig,FtUpwdDnwdMovConfig
  Bus Selector5 : BusSelector  OutputSignals=KeSMSuFirstRwStFwdBkwdPosDelta_Val,KeSMSuFirstRwStFootrestPosDelta_Val,KeSMSuFirstRwStBackPosDelta_Val
  CheckAtPos : Lib/CheckAtPos  SystemSampleTime=-1
  Constant : Constant  Value=0  OutDataTypeStr=boolean
  Constant1 : Constant  Value=0  OutDataTypeStr=boolean
  IsArrivedTarZone1 : Lib/CommonUsed/IniPosjudg/Subsystem2  SystemSampleTime=-1
  Drv_ArrivedTarPos : Outport
  wires:
  DrvCurPos/1 -> Bus Selector/1
  Bus Selector/4 -> [DrvStCshnRrUpwdDnwdPos]  "<IfVeSMSuDrvStCshnRrUpwdDnwdPos_Val_read>"
  Bus Selector/5 -> [DrvStFrwdBkwdPos]  "<IfVeSMSuDrvStFrwdBkwdPos_Val_read>"
  Bus Selector/2 -> [DrvStBkReclnUpwdDnwdPos]  "<IfVeSMSuDrvStBkReclnUpwdDnwdPos_Val_read>"
  Bus Selector/1 -> [DrvStFtUpwdDnwdPos]  "<IfVeSMSuDrvStFtUpwdDnwdPos_Val_read>"
  Bus Selector/3 -> [DrvStCshnFrntUpwdDnwdPos]  "<IfVeSMSuDrvStCshnFrntUpwdDnwdPos_Val_read>"
  Bus Selector2/2 -> [K_BkReclnUpwdDnwdPosMax]  "<BkReclnUpwdDnwdPosMax>"
  Bus Selector2/9 -> [K_FtUpwdDnwdPosMin]  "<FtUpwdDnwdPosMin>"
  Bus Selector3/1 -> Bus Selector2/1  "<RecvDrvSt>"
  ModeStCalib_Drv/1 -> Bus Selector3/1
  Bus Selector2/6 -> [K_FrwdBkwdPosMin]  "<FrwdBkwdPosMin>"
  Bus Selector2/3 -> [K_BkReclnUpwdDnwdPosMin]  "<BkReclnUpwdDnwdPosMin>"
  Bus Selector2/4 -> [K_FrwdBkwdPos]  "<FrwdBkwdPos>"
  Bus Selector2/7 -> [K_FtUpwdDnwdPos]  "<FtUpwdDnwdPos>"
  Bus Selector2/5 -> [K_FrwdBkwdPosMax]  "<FrwdBkwdPosMax>"
  Bus Selector2/1 -> [K_BkReclnUpwdDnwdPos]  "<BkReclnUpwdDnwdPos>"
  Bus Selector2/8 -> [K_FtUpwdDnwdPosMax]  "<FtUpwdDnwdPosMax>"
  DrvCurPosV/1 -> Bus Selector1/1
  Bus Selector1/3 -> [DrvStCshnFrntUpwdDnwdPosV]  "<IfVeSMSuDrvStCshnFrntUpwdDnwdPosV_Val_read>"
  Bus Selector1/2 -> [DrvStBkReclnUpwdDnwdPosV]  "<IfVeSMSuDrvStBkReclnUpwdDnwdPosV_Val_read>"
  Bus Selector1/1 -> [DrvStFtUpwdDnwdPosV]  "<IfVeSMSuDrvStFtUpwdDnwdPosV_Val_read>"
  Bus Selector1/4 -> [DrvStCshnRrUpwdDnwdPosV]  "<IfVeSMSuDrvStCshnRrUpwdDnwdPosV_Val_read>"
  Bus Selector1/5 -> [DrvStFrwdBkwdPosV]  "<IfVeSMSuDrvStFrwdBkwdPosV_Val_read>"
  [FtUpwdDnwdMovConfig] -> CheckAtPos/1
  [K_FtUpwdDnwdPosMax] -> IsArrivedTarZone1/4
  [KeSMSuFirstRwStFootrestPosDelta_Val] -> IsArrivedTarZone1/3
  [K_FtUpwdDnwdPosMin] -> IsArrivedTarZone1/2
  [DrvStFtUpwdDnwdPos] -> IsArrivedTarZone1/1
  Bus Selector4/3 -> [FtUpwdDnwdMovConfig]  "<FtUpwdDnwdMovConfig>"
  Bus Selector4/1 -> [BkReclnUpwdDnwdMovConfig]  "<BkReclnUpwdDnwdMovConfig>"
  Bus Selector4/2 -> [FrwdBkwdMovConfig]  "<FrwdBkwdMovConfig>"
  StConfig/1 -> Bus Selector4/1
  [DrvStFtUpwdDnwdPosV] -> CheckAtPos/2
  IsArrivedTarZone1/1 -> CheckAtPos/3
  CheckAtPos/1 -> Drv_ArrivedTarPos/1
  Constant/1 -> CheckAtPos/4
  Constant1/1 -> CheckAtPos/5
  PosDeltaCalib/1 -> Bus Selector5/1
  Bus Selector5/1 -> [KeSMSuFirstRwStBackPosDelta_Val]  "<KeSMSuFirstRwStFwdBkwdPosDelta_Val>"
  Bus Selector5/3 -> [KeSMSuFirstRwStFwdBkwdPosDelta_Val]  "<KeSMSuFirstRwStBackPosDelta_Val>"
  Bus Selector5/2 -> [KeSMSuFirstRwStFootrestPosDelta_Val]  "<KeSMSuFirstRwStFootrestPosDelta_Val>"

== system ModeAdjust/ModeAdjustRunnable_sys/ModeAdjust/ArrivedAtTargetPosChk/Recovery/Pass ==
  PassStPoss : Inport
  ModeStCalib_Pass : Inport  Port=2
  StConfig : Inport  Port=3
  PassStPossV : Inport  Port=4
  PosDeltaCalib : Inport  Port=5
  Bus Selector1 : BusSelector  OutputSignals=IfVeSMSuPassStBkReclnUpwdDnwdPos_Val_read,IfVeSMSuPassStCshnFrntUpwdDnwdPos_Val_read,IfVeSMSuPassStCshnRrUpwdDnwdPos_Val_read,IfVeSMSuPassStFrwdBkwdPos_Val_read,IfVeSMSuPassStFtUpwdDnwdPos_Val_read
  Bus Selector2 : BusSelector  OutputSignals=BkReclnUpwdDnwdPos,BkReclnUpwdDnwdPosMax,BkReclnUpwdDnwdPosMin,FrwdBkwdPos,FrwdBkwdPosMax,FrwdBkwdPosMin,FtUpwdDnwdPos,FtUpwdDnwdPosMax,FtUpwdDnwdPosMin
  Bus Selector3 : BusSelector  OutputSignals=RecvPassSt
  Bus Selector4 : BusSelector  OutputSignals=BkReclnUpwdDnwdMovConfig,FrwdBkwdMovConfig,FtUpwdDnwdMovConfig
  Bus Selector5 : BusSelector  OutputSignals=IfVeSMSuPassStBkReclnUpwdDnwdPosV_Val_read,IfVeSMSuPassStCshnFrntUpwdDnwdPosV_Val_read,IfVeSMSuPassStCshnRrUpwdDnwdPosV_Val_read,IfVeSMSuPassStFrwdBkwdPosV_Val_read,IfVeSMSuPassStFtUpwdDnwdPosV_Val_read
  Bus Selector6 : BusSelector  OutputSignals=KeSMSuFirstRwStFwdBkwdPosDelta_Val,KeSMSuFirstRwStFootrestPosDelta_Val,KeSMSuFirstRwStBackPosDelta_Val
  CheckAtPos : Lib/CheckAtPos  SystemSampleTime=-1
  Constant : Constant  Value=0  OutDataTypeStr=boolean
  Constant1 : Constant  Value=0  OutDataTypeStr=boolean
  IsArrivedTarZone1 : Lib/CommonUsed/IniPosjudg/Subsystem2  SystemSampleTime=-1
  Pass_ArrivedTarPos : Outport
  wires:
  [PassStFtUpwdDnwdPos] -> IsArrivedTarZone1/1
  IsArrivedTarZone1/1 -> [Step1_2_ArrivedTarPos]
  [K_FtUpwdDnwdPosMin] -> IsArrivedTarZone1/2
  [KeSMSuFirstRwStFootrestPosDelta_Val] -> IsArrivedTarZone1/3
  Bus Selector1/3 -> [PassStCshnRrUpwdDnwdPos]  "<IfVeSMSuPassStCshnRrUpwdDnwdPos_Val_read>"
  Bus Selector1/1 -> [PassStBkReclnUpwdDnwdPos]  "<IfVeSMSuPassStBkReclnUpwdDnwdPos_Val_read>"
  Bus Selector1/5 -> [PassStFtUpwdDnwdPos]  "<IfVeSMSuPassStFtUpwdDnwdPos_Val_read>"
  Bus Selector1/4 -> [PassStFrwdBkwdPos]  "<IfVeSMSuPassStFrwdBkwdPos_Val_read>"
  PassStPoss/1 -> Bus Selector1/1
  Bus Selector1/2 -> [PassStCshnFrntUpwdDnwdPos]  "<IfVeSMSuPassStCshnFrntUpwdDnwdPos_Val_read>"
  [K_FtUpwdDnwdPosMax] -> IsArrivedTarZone1/4
  Bus Selector2/2 -> [K_BkReclnUpwdDnwdPosMax]  "<BkReclnUpwdDnwdPosMax>"
  Bus Selector2/9 -> [K_FtUpwdDnwdPosMin]  "<FtUpwdDnwdPosMin>"
  Bus Selector3/1 -> Bus Selector2/1  "<RecvPassSt>"
  ModeStCalib_Pass/1 -> Bus Selector3/1
  Bus Selector2/6 -> [K_FrwdBkwdPosMin]  "<FrwdBkwdPosMin>"
  Bus Selector2/3 -> [K_BkReclnUpwdDnwdPosMin]  "<BkReclnUpwdDnwdPosMin>"
  Bus Selector2/4 -> [K_FrwdBkwdPos]  "<FrwdBkwdPos>"
  Bus Selector2/7 -> [K_FtUpwdDnwdPos]  "<FtUpwdDnwdPos>"
  Bus Selector2/5 -> [K_FrwdBkwdPosMax]  "<FrwdBkwdPosMax>"
  Bus Selector2/1 -> [K_BkReclnUpwdDnwdPos]  "<BkReclnUpwdDnwdPos>"
  Bus Selector2/8 -> [K_FtUpwdDnwdPosMax]  "<FtUpwdDnwdPosMax>"
  Bus Selector4/3 -> [FtUpwdDnwdMovConfig]  "<FtUpwdDnwdMovConfig>"
  StConfig/1 -> Bus Selector4/1
  Bus Selector4/2 -> [FrwdBkwdMovConfig]  "<FrwdBkwdMovConfig>"
  Bus Selector4/1 -> [BkReclnUpwdDnwdMovConfig]  "<BkReclnUpwdDnwdMovConfig>"
  Bus Selector5/3 -> [PassStCshnRrUpwdDnwdPosV]  "<IfVeSMSuPassStCshnRrUpwdDnwdPosV_Val_read>"
  Bus Selector5/2 -> [PassStCshnFrntUpwdDnwdPosV]  "<IfVeSMSuPassStCshnFrntUpwdDnwdPosV_Val_read>"
  Bus Selector5/5 -> [PassStFtUpwdDnwdPosV]  "<IfVeSMSuPassStFtUpwdDnwdPosV_Val_read>"
  Bus Selector5/1 -> [PassStBkReclnUpwdDnwdPosV]  "<IfVeSMSuPassStBkReclnUpwdDnwdPosV_Val_read>"
  Bus Selector5/4 -> [PassStFrwdBkwdPosV]  "<IfVeSMSuPassStFrwdBkwdPosV_Val_read>"
  PassStPossV/1 -> Bus Selector5/1
  [FtUpwdDnwdMovConfig] -> CheckAtPos/1
  [Step1_2_ArrivedTarPos] -> CheckAtPos/3
  [PassStFtUpwdDnwdPosV] -> CheckAtPos/2
  CheckAtPos/1 -> Pass_ArrivedTarPos/1
  Constant/1 -> CheckAtPos/4
  Constant1/1 -> CheckAtPos/5
  PosDeltaCalib/1 -> Bus Selector6/1
  Bus Selector6/1 -> [KeSMSuFirstRwStBackPosDelta_Val]  "<KeSMSuFirstRwStFwdBkwdPosDelta_Val>"
  Bus Selector6/3 -> [KeSMSuFirstRwStFwdBkwdPosDelta_Val]  "<KeSMSuFirstRwStBackPosDelta_Val>"
  Bus Selector6/2 -> [KeSMSuFirstRwStFootrestPosDelta_Val]  "<KeSMSuFirstRwStFootrestPosDelta_Val>"

== system ModeAdjust/ModeAdjustRunnable_sys/ModeAdjust/ArrivedAtTargetPosChk/Recovery/R2Lt ==
  SecRwLtStsPoss : Inport
  ModeStCalib_2L : Inport  Port=2
  StConfig : Inport  Port=3
  SecRwLtStPossV : Inport  Port=4
  PosDeltaCalib : Inport  Port=5
  Bus Selector : BusSelector  OutputSignals=IfVeSMSuSecRwLtStBkReclnUpwdDnwdPos_Val_read,IfVeSMSuSecRwLtStFrwdBkwdPos_Val_read,IfVeSMSuSecRwLtStHPassStUpwdDnwdPos_Val_read,IfVeSMSuSecRwLtStLgrstUpwdDnwdPos_Val_read,IfVeSMSuSecRwLtStLtwdRtwdPos_Val_read,IfVeSMSuSecRwLtStArmScrnPos_Val_read
  Bus Selector1 : BusSelector  OutputSignals=IfVeSMSuSecRwLtStBkReclnUpwdDnwdPosV_Val_read,IfVeSMSuSecRwLtStFrwdBkwdPosV_Val_read,IfVeSMSuSecRwLtStHPassStUpwdDnwdPosV_Val_read,IfVeSMSuSecRwLtStLgrstUpwdDnwdPosV_Val_read,IfVeSMSuSecRwLtStLtwdRtwdPosV_Val_read,IfVeSMSuSecRwLtStArmScrnPosV_Val_read
  Bus Selector2 : BusSelector  OutputSignals=ArmScrnPos,ArmScrnPosMax,ArmScrnPosMin,BkReclnUpwdDnwdPos,BkReclnUpwdDnwdPosMax,BkReclnUpwdDnwdPosMin,FrwdBkwdPos,FrwdBkwdPosMax,FrwdBkwdPosMin,HdrstUpwdPos,HdrstUpwdPosMax,HdrstUpwdPosMin,LgrstUpwdPos,LgrstUpwdPosMax,LgrstUpwdPosMin,LtwdRtwdPos,LtwdRtwdPosMax,LtwdRtwdPosMin
  Bus Selector3 : BusSelector  OutputSignals=RecoveryMdSecRwLtSt
  Bus Selector4 : BusSelector  OutputSignals=BkReclnUpwdDnwdMovConfig,ArmTouchMovConfig,FrwdBkwdMovConfig,LgrstUpwdMovConfig,LtwdRtwdMovConfig
  Bus Selector5 : BusSelector  OutputSignals=KeSMSuSecRwStArmTochPosDelta_Val,KeSMSuSecRwStBackPosDelta_Val,KeSMSuSecRwStFwdBkwdPosDelta_Val,KeSMSuSecRwStLegrestUpwdDwnwdPosDelta_Val,KeSMSuSecRwStLwdRwdPosDelta_Val
  CheckAtPos : Lib/CheckAtPos  SystemSampleTime=-1
  CheckAtPos1 : Lib/CheckAtPos  SystemSampleTime=-1
  Constant{,1..3} (4 alike) : Constant  Value=0  OutDataTypeStr=boolean
  IsArrivedTarZone : Lib/CommonUsed/IniPosjudg/Subsystem2  SystemSampleTime=-1
  IsArrivedTarZone1 : Lib/CommonUsed/IniPosjudg/Subsystem2  SystemSampleTime=-1
  Logical Operator9 : Logic  AllPortsSameDT=off  OutDataTypeStr=boolean
  R2Lt_ArrivedTarPos : Outport
  wires:
  IsArrivedTarZone/1 -> [Step1_1_ArrivedTarPos]
  [SecRwLtStBkReclnUpwdDnwdPos] -> IsArrivedTarZone/1
  [K_BkReclnUpwdDnwdPosMin] -> IsArrivedTarZone/2
  Bus Selector/5 -> [SecRwLtStLtwdRtwdPos]  "<IfVeSMSuSecRwLtStLtwdRtwdPos_Val_read>"
  SecRwLtStsPoss/1 -> Bus Selector/1
  Bus Selector/3 -> [SecRwLtStHPassStUpwdDnwdPos]  "<IfVeSMSuSecRwLtStHPassStUpwdDnwdPos_Val_read>"
  Bus Selector/4 -> [SecRwLtStLgrstUpwdDnwdPos]  "<IfVeSMSuSecRwLtStLgrstUpwdDnwdPos_Val_read>"
  Bus Selector/2 -> [SecRwLtStFrwdBkwdPos]  "<IfVeSMSuSecRwLtStFrwdBkwdPos_Val_read>"
  Bus Selector/1 -> [SecRwLtStBkReclnUpwdDnwdPos]  "<IfVeSMSuSecRwLtStBkReclnUpwdDnwdPos_Val_read>"
  [K_LgrstUpwdPosMin] -> IsArrivedTarZone1/2
  [SecRwLtStLgrstUpwdDnwdPos] -> IsArrivedTarZone1/1
  IsArrivedTarZone1/1 -> [Step1_2_ArrivedTarPos]
  Logical Operator9/1 -> R2Lt_ArrivedTarPos/1
  Bus Selector/6 -> [SecRwLtStArmScrnPos]  "<IfVeSMSuSecRwLtStArmScrnPos_Val_read>"
  [KeSMSuSecRwStBackPosDelta_Val] -> IsArrivedTarZone/3
  [K_BkReclnUpwdDnwdPosMax] -> IsArrivedTarZone/4
  [K_LgrstUpwdPosMax] -> IsArrivedTarZone1/4
  [KeSMSuSecRwStLegrestUpwdDwnwdPosDelta_Val] -> IsArrivedTarZone1/3
  Bus Selector2/1 -> [K_ArmScrnPos]  "<ArmScrnPos>"
  Bus Selector2/18 -> [K_LtwdRtwdPosMin]  "<LtwdRtwdPosMin>"
  Bus Selector2/16 -> [K_LtwdRtwdPos]  "<LtwdRtwdPos>"
  Bus Selector2/15 -> [K_LgrstUpwdPosMin]  "<LgrstUpwdPosMin>"
  Bus Selector2/17 -> [K_LtwdRtwdPosMax]  "<LtwdRtwdPosMax>"
  Bus Selector2/12 -> [K_HdrstUpwdPosMin]  "<HdrstUpwdPosMin>"
  Bus Selector2/13 -> [K_LgrstUpwdPos]  "<LgrstUpwdPos>"
  Bus Selector2/11 -> [K_HdrstUpwdPosMax]  "<HdrstUpwdPosMax>"
  Bus Selector2/14 -> [K_LgrstUpwdPosMax]  "<LgrstUpwdPosMax>"
  Bus Selector2/10 -> [K_HdrstUpwdPos]  "<HdrstUpwdPos>"
  Bus Selector2/4 -> [K_BkReclnUpwdDnwdPos]  "<BkReclnUpwdDnwdPos>"
  Bus Selector2/9 -> [K_FrwdBkwdPosMin]  "<FrwdBkwdPosMin>"
  Bus Selector2/5 -> [K_BkReclnUpwdDnwdPosMax]  "<BkReclnUpwdDnwdPosMax>"
  Bus Selector2/8 -> [K_FrwdBkwdPosMax]  "<FrwdBkwdPosMax>"
  Bus Selector3/1 -> Bus Selector2/1  "<RecoveryMdSecRwLtSt>"
  Bus Selector2/7 -> [K_FrwdBkwdPos]  "<FrwdBkwdPos>"
  Bus Selector2/3 -> [K_ArmScrnPosMin]  "<ArmScrnPosMin>"
  Bus Selector2/2 -> [K_ArmScrnPosMax]  "<ArmScrnPosMax>"
  Bus Selector2/6 -> [K_BkReclnUpwdDnwdPosMin]  "<BkReclnUpwdDnwdPosMin>"
  ModeStCalib_2L/1 -> Bus Selector3/1
  StConfig/1 -> Bus Selector4/1
  Bus Selector4/3 -> [FrwdBkwdMovConfig]  "<FrwdBkwdMovConfig>"
  Bus Selector4/5 -> [LtwdRtwdMovConfig]  "<LtwdRtwdMovConfig>"
  Bus Selector4/4 -> [LgrstUpwdMovConfig]  "<LgrstUpwdMovConfig>"
  Bus Selector4/2 -> [ArmTouchMovConfig]  "<ArmTouchMovConfig>"
  Bus Selector4/1 -> [BkReclnUpwdDnwdMovConfig]  "<BkReclnUpwdDnwdMovConfig>"
  SecRwLtStPossV/1 -> Bus Selector1/1
  Bus Selector1/4 -> [SecRwLtStLgrstUpwdDnwdPosV]  "<IfVeSMSuSecRwLtStLgrstUpwdDnwdPosV_Val_read>"
  Bus Selector1/1 -> [SecRwLtStBkReclnUpwdDnwdPosV]  "<IfVeSMSuSecRwLtStBkReclnUpwdDnwdPosV_Val_read>"
  Bus Selector1/2 -> [SecRwLtStFrwdBkwdPosV]  "<IfVeSMSuSecRwLtStFrwdBkwdPosV_Val_read>"
  Bus Selector1/3 -> [SecRwLtStHPassStUpwdDnwdPosV]  "<IfVeSMSuSecRwLtStHPassStUpwdDnwdPosV_Val_read>"
  Bus Selector1/5 -> [SecRwLtStLtwdRtwdPosV]  "<IfVeSMSuSecRwLtStLtwdRtwdPosV_Val_read>"
  Bus Selector1/6 -> [IfVeSMSuSecRwLtStArmScrnPosV]  "<IfVeSMSuSecRwLtStArmScrnPosV_Val_read>"
  [BkReclnUpwdDnwdMovConfig] -> CheckAtPos/1
  [Step1_1_ArrivedTarPos] -> CheckAtPos/3
  [LgrstUpwdMovConfig] -> CheckAtPos1/1
  [Step1_2_ArrivedTarPos] -> CheckAtPos1/3
  CheckAtPos1/1 -> Logical Operator9/2
  CheckAtPos/1 -> Logical Operator9/1
  [SecRwLtStBkReclnUpwdDnwdPosV] -> CheckAtPos/2
  [SecRwLtStLgrstUpwdDnwdPosV] -> CheckAtPos1/2
  Constant/1 -> CheckAtPos/4
  Constant1/1 -> CheckAtPos/5
  Constant2/1 -> CheckAtPos1/4
  Constant3/1 -> CheckAtPos1/5
  Bus Selector5/5 -> [KeSMSuSecRwStLwdRwdPosDelta_Val]  "<KeSMSuSecRwStLwdRwdPosDelta_Val>"
  PosDeltaCalib/1 -> Bus Selector5/1
  Bus Selector5/2 -> [KeSMSuSecRwStBackPosDelta_Val]  "<KeSMSuSecRwStBackPosDelta_Val>"
  Bus Selector5/4 -> [KeSMSuSecRwStLegrestUpwdDwnwdPosDelta_Val]  "<KeSMSuSecRwStLegrestUpwdDwnwdPosDelta_Val>"
  Bus Selector5/1 -> [KeSMSuSecRwStArmTochPosDelta_Val]  "<KeSMSuSecRwStArmTochPosDelta_Val>"
  Bus Selector5/3 -> [KeSMSuSecRwStFwdBkwdPosDelta_Val]  "<KeSMSuSecRwStFwdBkwdPosDelta_Val>"

== system ModeAdjust/ModeAdjustRunnable_sys/ModeAdjust/ArrivedAtTargetPosChk/Recovery/R2Rt ==
  SecRwRtStPoss : Inport
  ModeStCalib_2R : Inport  Port=2
  StConfig : Inport  Port=3
  SecRwRtStPossV : Inport  Port=4
  PosDeltaCalib : Inport  Port=5
  Bus Selector : BusSelector  OutputSignals=IfVeSMSuSecRwRtStBkReclnUpwdDnwdPos_Val_read,IfVeSMSuSecRwRtStFrwdBkwdPos_Val_read,IfVeSMSuSecRwRtStHPassStUpwdDnwdPos_Val_read,IfVeSMSuSecRwRtStLgrstUpwdDnwdPos_Val_read,IfVeSMSuSecRwRtStLtwdRtwdPos_Val_read,SecRwRtStArmScrnPos_Val_read
  Bus Selector1 : BusSelector  OutputSignals=IfVeSMSuSecRwRtStBkReclnUpwdDnwdPosV_Val_read,IfVeSMSuSecRwRtStFrwdBkwdPosV_Val_read,IfVeSMSuSecRwRtStHPassStUpwdDnwdPosV_Val_read,IfVeSMSuSecRwRtStLgrstUpwdDnwdPosV_Val_read,IfVeSMSuSecRwRtStLtwdRtwdPosV_Val_read,SecRwRtStArmScrnPosV_Val_read
  Bus Selector2 : BusSelector  OutputSignals=ArmScrnPos,ArmScrnPosMax,ArmScrnPosMin,BkReclnUpwdDnwdPos,BkReclnUpwdDnwdPosMax,BkReclnUpwdDnwdPosMin,FrwdBkwdPos,FrwdBkwdPosMax,FrwdBkwdPosMin,HdrstUpwdPos,HdrstUpwdPosMax,HdrstUpwdPosMin,LgrstUpwdPos,LgrstUpwdPosMax,LgrstUpwdPosMin,LtwdRtwdPos,LtwdRtwdPosMax,LtwdRtwdPosMin
  Bus Selector3 : BusSelector  OutputSignals=RecoveryMdSecRwRtSt
  Bus Selector4 : BusSelector  OutputSignals=BkReclnUpwdDnwdMovConfig,ArmTouchMovConfig,FrwdBkwdMovConfig,LgrstUpwdMovConfig,LtwdRtwdMovConfig
  Bus Selector5 : BusSelector  OutputSignals=KeSMSuSecRwStArmTochPosDelta_Val,KeSMSuSecRwStBackPosDelta_Val,KeSMSuSecRwStFwdBkwdPosDelta_Val,KeSMSuSecRwStLegrestUpwdDwnwdPosDelta_Val,KeSMSuSecRwStLwdRwdPosDelta_Val
  CheckAtPos : Lib/CheckAtPos  SystemSampleTime=-1
  CheckAtPos1 : Lib/CheckAtPos  SystemSampleTime=-1
  Constant{1..4} (4 alike) : Constant  Value=0  OutDataTypeStr=boolean
  IsArrivedTarZone : Lib/CommonUsed/IniPosjudg/Subsystem2  SystemSampleTime=-1
  IsArrivedTarZone1 : Lib/CommonUsed/IniPosjudg/Subsystem2  SystemSampleTime=-1
  Logical Operator9 : Logic  AllPortsSameDT=off  OutDataTypeStr=boolean
  R2Rt_ArrivedTarPos : Outport
  wires:
  IsArrivedTarZone1/1 -> [Step1_2_ArrivedTarPos]
  [SecRwRtStLgrstUpwdDnwdPos] -> IsArrivedTarZone1/1
  [K_LgrstUpwdPosMin] -> IsArrivedTarZone1/2
  [K_BkReclnUpwdDnwdPosMin] -> IsArrivedTarZone/2
  [SecRwRtStBkReclnUpwdDnwdPos] -> IsArrivedTarZone/1
  IsArrivedTarZone/1 -> [Step1_1_ArrivedTarPos]
  Bus Selector/4 -> [SecRwRtStLgrstUpwdDnwdPos]  "<IfVeSMSuSecRwRtStLgrstUpwdDnwdPos_Val_read>"
  Bus Selector/1 -> [SecRwRtStBkReclnUpwdDnwdPos]  "<IfVeSMSuSecRwRtStBkReclnUpwdDnwdPos_Val_read>"
  Bus Selector/5 -> [SecRwRtStLtwdRtwdPos]  "<IfVeSMSuSecRwRtStLtwdRtwdPos_Val_read>"
  SecRwRtStPoss/1 -> Bus Selector/1
  Bus Selector/3 -> [SecRwRtStHPassStUpwdDnwdPos]  "<IfVeSMSuSecRwRtStHPassStUpwdDnwdPos_Val_read>"
  Bus Selector/2 -> [SecRwRtStFrwdBkwdPos]  "<IfVeSMSuSecRwRtStFrwdBkwdPos_Val_read>"
  Logical Operator9/1 -> R2Rt_ArrivedTarPos/1
  Bus Selector/6 -> [SecRwRtStArmScrnPos]  "<SecRwRtStArmScrnPos_Val_read>"
  [KeSMSuSecRwStBackPosDelta_Val] -> IsArrivedTarZone/3
  [KeSMSuSecRwStLegrestUpwdDwnwdPosDelta_Val] -> IsArrivedTarZone1/3
  [K_BkReclnUpwdDnwdPosMax] -> IsArrivedTarZone/4
  [K_LgrstUpwdPosMax] -> IsArrivedTarZone1/4
  Bus Selector2/1 -> [K_ArmScrnPos]  "<ArmScrnPos>"
  Bus Selector2/18 -> [K_LtwdRtwdPosMin]  "<LtwdRtwdPosMin>"
  Bus Selector2/16 -> [K_LtwdRtwdPos]  "<LtwdRtwdPos>"
  Bus Selector2/15 -> [K_LgrstUpwdPosMin]  "<LgrstUpwdPosMin>"
  Bus Selector2/17 -> [K_LtwdRtwdPosMax]  "<LtwdRtwdPosMax>"
  Bus Selector2/12 -> [K_HdrstUpwdPosMin]  "<HdrstUpwdPosMin>"
  Bus Selector2/13 -> [K_LgrstUpwdPos]  "<LgrstUpwdPos>"
  Bus Selector2/11 -> [K_HdrstUpwdPosMax]  "<HdrstUpwdPosMax>"
  Bus Selector2/14 -> [K_LgrstUpwdPosMax]  "<LgrstUpwdPosMax>"
  Bus Selector2/10 -> [K_HdrstUpwdPos]  "<HdrstUpwdPos>"
  Bus Selector2/4 -> [K_BkReclnUpwdDnwdPos]  "<BkReclnUpwdDnwdPos>"
  Bus Selector2/9 -> [K_FrwdBkwdPosMin]  "<FrwdBkwdPosMin>"
  Bus Selector2/5 -> [K_BkReclnUpwdDnwdPosMax]  "<BkReclnUpwdDnwdPosMax>"
  Bus Selector2/8 -> [K_FrwdBkwdPosMax]  "<FrwdBkwdPosMax>"
  Bus Selector3/1 -> Bus Selector2/1  "<RecoveryMdSecRwRtSt>"
  Bus Selector2/7 -> [K_FrwdBkwdPos]  "<FrwdBkwdPos>"
  Bus Selector2/3 -> [K_ArmScrnPosMin]  "<ArmScrnPosMin>"
  Bus Selector2/2 -> [K_ArmScrnPosMax]  "<ArmScrnPosMax>"
  Bus Selector2/6 -> [K_BkReclnUpwdDnwdPosMin]  "<BkReclnUpwdDnwdPosMin>"
  ModeStCalib_2R/1 -> Bus Selector3/1
  StConfig/1 -> Bus Selector4/1
  Bus Selector4/3 -> [FrwdBkwdMovConfig]  "<FrwdBkwdMovConfig>"
  Bus Selector4/5 -> [LtwdRtwdMovConfig]  "<LtwdRtwdMovConfig>"
  Bus Selector4/4 -> [LgrstUpwdMovConfig]  "<LgrstUpwdMovConfig>"
  Bus Selector4/2 -> [ArmTouchMovConfig]  "<ArmTouchMovConfig>"
  Bus Selector4/1 -> [BkReclnUpwdDnwdMovConfig]  "<BkReclnUpwdDnwdMovConfig>"
  Bus Selector1/1 -> [SecRwRtStBkReclnUpwdDnwdPosV]  "<IfVeSMSuSecRwRtStBkReclnUpwdDnwdPosV_Val_read>"
  Bus Selector1/5 -> [SecRwRtStLtwdRtwdPosV]  "<IfVeSMSuSecRwRtStLtwdRtwdPosV_Val_read>"
  Bus Selector1/4 -> [SecRwRtStLgrstUpwdDnwdPosV]  "<IfVeSMSuSecRwRtStLgrstUpwdDnwdPosV_Val_read>"
  Bus Selector1/6 -> [SecRwRtStArmScrnPosV]  "<SecRwRtStArmScrnPosV_Val_read>"
  SecRwRtStPossV/1 -> Bus Selector1/1
  Bus Selector1/3 -> [SecRwRtStHPassStUpwdDnwdPosV]  "<IfVeSMSuSecRwRtStHPassStUpwdDnwdPosV_Val_read>"
  Bus Selector1/2 -> [SecRwRtStFrwdBkwdPosV]  "<IfVeSMSuSecRwRtStFrwdBkwdPosV_Val_read>"
  CheckAtPos1/1 -> Logical Operator9/2
  CheckAtPos/1 -> Logical Operator9/1
  [BkReclnUpwdDnwdMovConfig] -> CheckAtPos/1
  [Step1_1_ArrivedTarPos] -> CheckAtPos/3
  [LgrstUpwdMovConfig] -> CheckAtPos1/1
  [Step1_2_ArrivedTarPos] -> CheckAtPos1/3
  [SecRwRtStBkReclnUpwdDnwdPosV] -> CheckAtPos/2
  [SecRwRtStLgrstUpwdDnwdPosV] -> CheckAtPos1/2
  Constant3/1 -> CheckAtPos/5
  Constant2/1 -> CheckAtPos/4
  Constant4/1 -> CheckAtPos1/5
  Constant1/1 -> CheckAtPos1/4
  Bus Selector5/5 -> [KeSMSuSecRwStLwdRwdPosDelta_Val]  "<KeSMSuSecRwStLwdRwdPosDelta_Val>"
  PosDeltaCalib/1 -> Bus Selector5/1
  Bus Selector5/2 -> [KeSMSuSecRwStBackPosDelta_Val]  "<KeSMSuSecRwStBackPosDelta_Val>"
  Bus Selector5/4 -> [KeSMSuSecRwStLegrestUpwdDwnwdPosDelta_Val]  "<KeSMSuSecRwStLegrestUpwdDwnwdPosDelta_Val>"
  Bus Selector5/1 -> [KeSMSuSecRwStArmTochPosDelta_Val]  "<KeSMSuSecRwStArmTochPosDelta_Val>"
  Bus Selector5/3 -> [KeSMSuSecRwStFwdBkwdPosDelta_Val]  "<KeSMSuSecRwStFwdBkwdPosDelta_Val>"
